simulink model "base_model"  (R2023b)
settings: Solver=ode3  StartTime=0.0  StopTime=5  FixedStep=0.001  RelTol=1e-3
libraries: cstblocks x1
settings Model: Creator=PC  LastModifiedBy=ASUS
settings DebuggingCC: UnconnectedInputMsg=warning  UnconnectedOutputMsg=warning  UnconnectedLineMsg=warning
settings ModelReferenceCC: EnableRefExpFcnMdlSchedulingChecks=on
settings RTWCC: DLArmComputeVersion=19.05

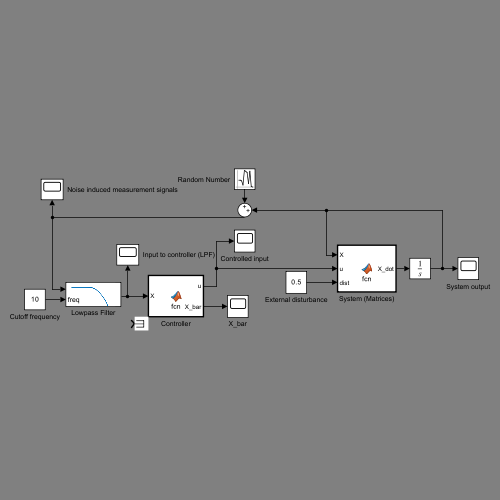
[thumbnail: Simulink's stored preview of the top-level diagram]
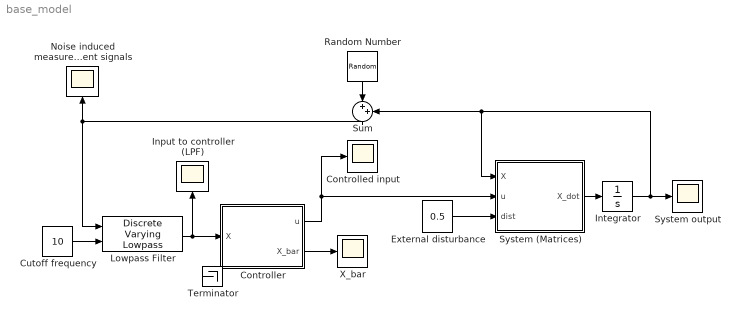
== system base_model ==
  Controlled input : Scope
  Controller : MATLAB Function  TreatAsAtomicUnit=on
  Cutoff frequency : Constant  Value=10  SampleTime=0.001
  External disturbance : Constant  Value=0.5  SampleTime=0.001
  Input to controller (LPF) : Scope
  Integrator : Integrator  InitialCondition=[0;-2;0 ; 4; 0; 5]
  Lowpass Filter : cstblocks/Linear Parameter Varying/Discrete Varying Lowpass  N=1  w0=0  Ts=0.01
  Noise induced measurement signals : Scope
  Random Number : RandomNumber  Variance=0.001  SampleTime=0.001
  Sum : Sum  Inputs=|++
  System (Matrices) : MATLAB Function  TreatAsAtomicUnit=on
  System output : Scope
  Terminator : Terminator
  X_bar : Scope
  wires:
  Controller/1(u) -> Controlled input/1, System (Matrices)/2(u)
  System (Matrices)/1(X_dot) -> Integrator/1
  Controller/2(X_bar) -> X_bar/1
  Integrator/1 -> System output/1, Sum/2, System (Matrices)/1(X)
  Cutoff frequency/1 -> Lowpass Filter/2
  Lowpass Filter/1 -> Controller/1(X), Input to controller (LPF)/1
  Sum/1 -> Lowpass Filter/1, Noise induced measurement signals/1
  Random Number/1 -> Sum/1
  External disturbance/1 -> System (Matrices)/3(dist)

== matlab function base_model/Controller ==
  data: X input; u output; X_bar output
function [u,X_bar] = fcn(X)
G=6.673*(10.^(-11));
M=6*10^24;
R=500000;
w = sqrt(G*M/(R^3));
x_CT = X(1);
y_CT = X(2);
z_CT = X(3);
x_CT_dot = X(4);
y_CT_dot = X(5);
z_CT_dot = X(6);
Kx = 2;
Ky = 2;                                % Kx, Ky, Kz=0 is a bad idea, it doesn't even control
Kz = 2;                                %increasing Kx, Ky, Kz increases peak overshoot
K = 10*eye(3);                         %what is K and Kx,y,z doing? what is the difference?
x_bar_CT = x_CT_dot + Kx*x_CT;
y_bar_CT = y_CT_dot + Ky*y_CT;
z_bar_CT = z_CT_dot + Kz*z_CT;
f_X = [(Kx*x_CT_dot) + (2*w*y_CT_dot) + (3*(w.^2)*x_CT);(Ky*y_CT_dot) - (2*w*x_CT_dot);(Kz*z_CT_dot) - ((w.^2)*z_CT)];
g_X = 2*eye(3);                        %decreasing the constant increases oscillations, increasing the same decreases the oscillations
X_bar = [x_bar_CT;y_bar_CT;z_bar_CT]; 
u = inv(g_X)*(-f_X - K*X_bar);

== matlab function base_model/System (Matrices) ==
  data: X input; u input; X_dot output; dist input
function X_dot  = fcn(X,u,dist)
G=6.673*(10.^(-11));
M=6*10^24;
R=500000;
w = sqrt(G*M/(R^3));
A=[0 0 0 1 0 0; 0 0 0 0 1 0; 0 0 0 0 0 1; 3*w*w 0 0 0 2*w 0; 0 0 0 -2*w 0 0;0 0 -w*w 0 0 0];
B=[0 0 0;0 0 0;0 0 0;2 0 0; 0 2 0; 0 0 2];
C=[1 0 0 0 0 0; 0 1 0 0 0 0;0 0 1 0 0 0];
X_dot = A*X + B*u + dist.*[0;0;0;1;1;1];
